simulink model "BassengreguleringSimulink"  (R2023a)
settings: Solver=VariableStepAuto  StartTime=0.0  StopTime=3600*142  RelTol=1e-3
values from neighbouring files (symbols this model uses):
  C = 4184 * 54000    (= 225936000)    [bassengregulering.m]
  k = 350    [bassengregulering.m]
  ki = 0.007    [bassengregulering.m]
  kp = 10000    [bassengregulering.m]
settings Model: Creator=odins  LastModifiedBy=augus

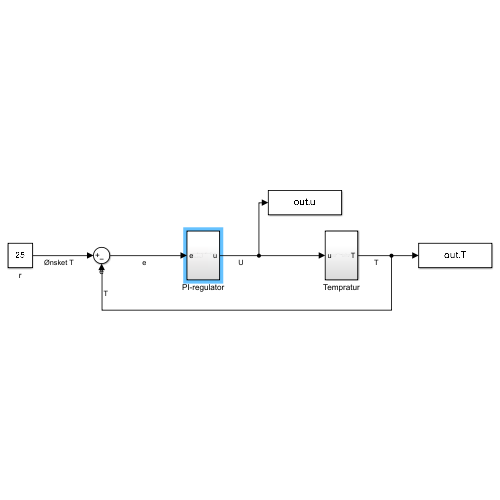
[thumbnail: Simulink's stored preview of the top-level diagram]
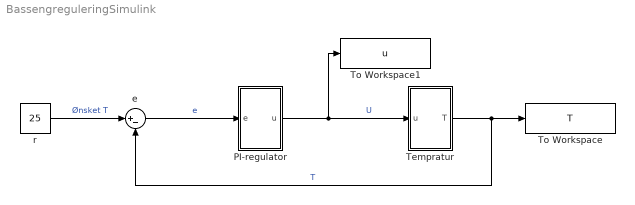
== system BassengreguleringSimulink ==
  PI-regulator : Subsystem
  Tempratur : Subsystem
  To Workspace : ToWorkspace  VariableName=T  SaveFormat=Timeseries  SampleTime=-1
  To Workspace1 : ToWorkspace  VariableName=u  SaveFormat=Timeseries  SampleTime=-1
  e : Sum  Inputs=|+-
  r : Constant  Value=25
  wires:
  r/1 -> e/1  "Ønsket T"
  PI-regulator/1(u) -> To Workspace1/1, Tempratur/1(u)  "U"
  e/1 -> PI-regulator/1(e)  "e"
  Tempratur/1(T) -> To Workspace/1, e/2  "T"

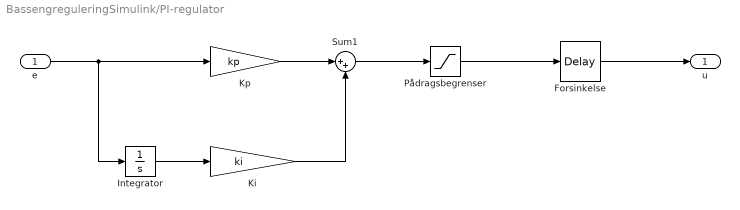
== system BassengreguleringSimulink/PI-regulator ==
  e : Inport
  Forsinkelse : TransportDelay  DelayTime=60
  Integrator : Integrator
  Ki : Gain  Gain=ki
  Kp : Gain  Gain=kp
  Pådragsbegrenser : Saturate  UpperLimit=36000  LowerLimit=0
  Sum1 : Sum  Inputs=|++
  u : Outport
  wires:
  Pådragsbegrenser/1 -> Forsinkelse/1
  Kp/1 -> Sum1/1
  Forsinkelse/1 -> u/1
  Integrator/1 -> Ki/1
  e/1 -> Integrator/1, Kp/1
  Sum1/1 -> Pådragsbegrenser/1
  Ki/1 -> Sum1/2

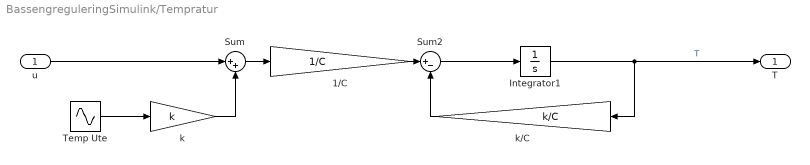
== system BassengreguleringSimulink/Tempratur ==
  u : Inport
  1/C : Gain  Gain=1/C
  Integrator1 : Integrator  InitialCondition=10
  Sum : Sum  Inputs=|++
  Sum2 : Sum  Inputs=|+-
  Temp Ute : Sin  Amplitude=5  Bias=10  Frequency=3.2/86400  SampleTime=0
  k : Gain  Gain=k
  k/C : Gain  Gain=k/C
  T : Outport
  wires:
  Sum2/1 -> Integrator1/1
  Temp Ute/1 -> k/1
  k/1 -> Sum/2
  Sum/1 -> 1/C/1
  1/C/1 -> Sum2/1
  k/C/1 -> Sum2/2
  Integrator1/1 -> T/1, k/C/1  "T"
  u/1 -> Sum/1
